simulink model "straightcontrol1_francesco"  (R2025b)
settings: Solver=VariableStepAuto  StartTime=0.0  StopTime=20  MaxStep=0.01  RelTol=1e-3
settings Model: Creator=utente  LastModifiedBy=Utente

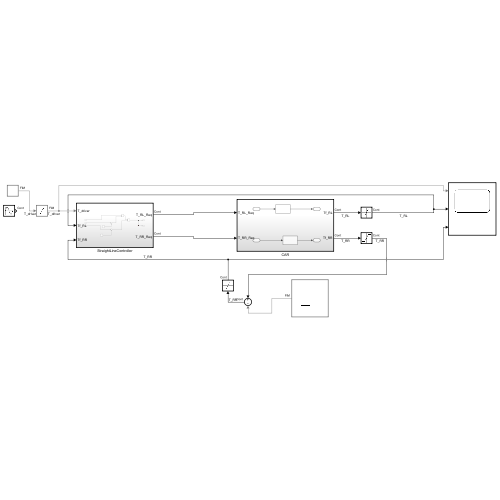
[thumbnail: Simulink's stored preview of the top-level diagram]
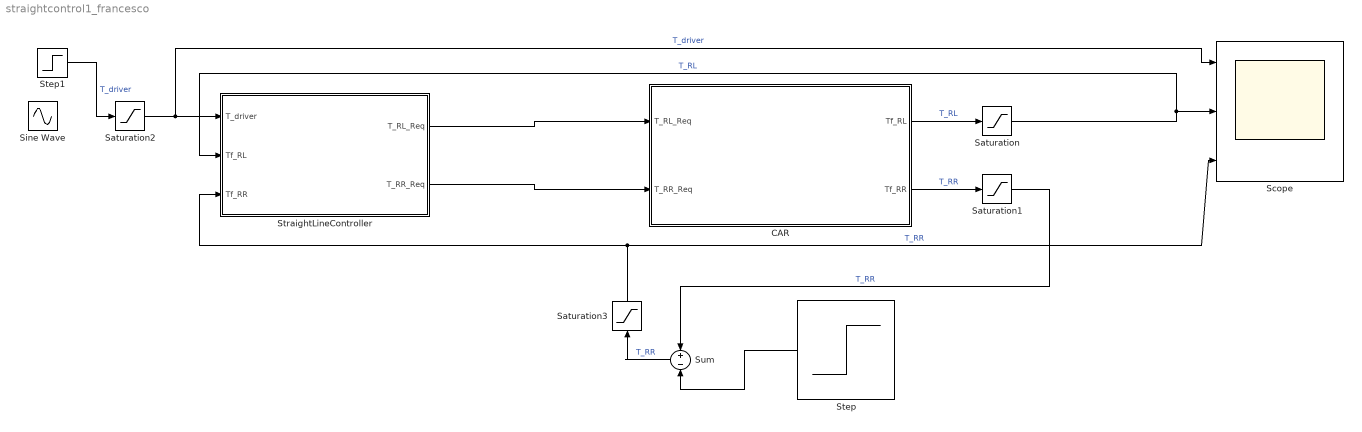
== system straightcontrol1_francesco ==
  CAR : Subsystem
  Saturation : Saturate  UpperLimit=21  LowerLimit=-21
  Saturation1 : Saturate  UpperLimit=21  LowerLimit=-21
  Saturation2 : Saturate  UpperLimit=21  LowerLimit=0
  Saturation3 : Saturate  UpperLimit=21  LowerLimit=0
  Scope : Scope  NumInputPorts=3
      settings: ActiveDisplayYMinimum=-1.1250000000000024  ActiveDisplayYMaximum=10.125000000000025
  Sine Wave : Sin  Amplitude=21  SampleTime=0
  Step : Step  Time=10  After=10  SampleTime=0
  Step1 : Step  After=21  SampleTime=0
  StraightLineController : Subsystem
  Sum : Sum  Inputs=+-
  wires:
  StraightLineController/1(T_RL_Req) -> CAR/1(T_RL_Req)
  StraightLineController/2(T_RR_Req) -> CAR/2(T_RR_Req)
  Step/1 -> Sum/2
  CAR/2(Tf_RR) -> Saturation1/1  "T_RR"
  CAR/1(Tf_RL) -> Saturation/1  "T_RL"
  Sum/1 -> Saturation3/1  "T_RR"
  Step1/1 -> Saturation2/1  "T_driver"
  Saturation/1 -> StraightLineController/2(Tf_RL), Scope/2  "T_RL"
  Saturation1/1 -> Sum/1  "T_RR"
  Saturation2/1 -> Scope/1, StraightLineController/1(T_driver)  "T_driver"
  Saturation3/1 -> StraightLineController/3(Tf_RR), Scope/3  "T_RR"

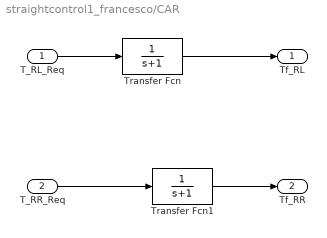
== system straightcontrol1_francesco/CAR ==
  T_RL_Req : Inport
  T_RR_Req : Inport  Port=2
  Transfer Fcn : TransferFcn  Denominator=[1 1]
  Transfer Fcn1 : TransferFcn  Denominator=[1 1]
  Tf_RL : Outport
  Tf_RR : Outport  Port=2
  wires:
  T_RL_Req/1 -> Transfer Fcn/1
  Transfer Fcn/1 -> Tf_RL/1
  Transfer Fcn1/1 -> Tf_RR/1
  T_RR_Req/1 -> Transfer Fcn1/1

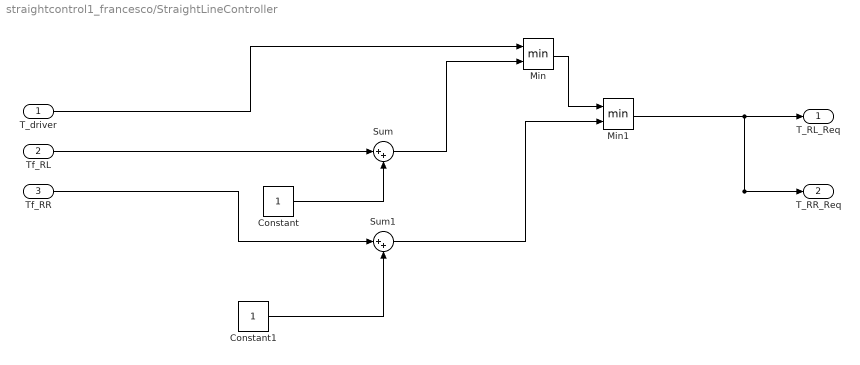
== system straightcontrol1_francesco/StraightLineController ==
  T_driver : Inport
  Tf_RL : Inport  Port=2
  Tf_RR : Inport  Port=3
  Constant : Constant
  Constant1 : Constant
  Min : MinMax  Inputs=2
  Min1 : MinMax  Inputs=2
  Sum : Sum  Inputs=|++
  Sum1 : Sum  Inputs=|++
  T_RL_Req : Outport
  T_RR_Req : Outport  Port=2
  wires:
  Sum/1 -> Min/2
  T_driver/1 -> Min/1
  Tf_RL/1 -> Sum/1
  Constant/1 -> Sum/2
  Tf_RR/1 -> Sum1/1
  Constant1/1 -> Sum1/2
  Min/1 -> Min1/1
  Sum1/1 -> Min1/2
  Min1/1 -> T_RR_Req/1, T_RL_Req/1
